simulink model "mdl_tubing_delays"  (R2020b)
settings: Solver=ode4  StartTime=0.0  StopTime=100  FixedStep=1e-3  RelTol=1e-3
undefined symbols (not defined in the file): m, n
libraries: simulink x2, sldelib x1, dspbuff3 x1
settings Model: EnablePacing=on  Creator=natha  LastModifiedBy=natha

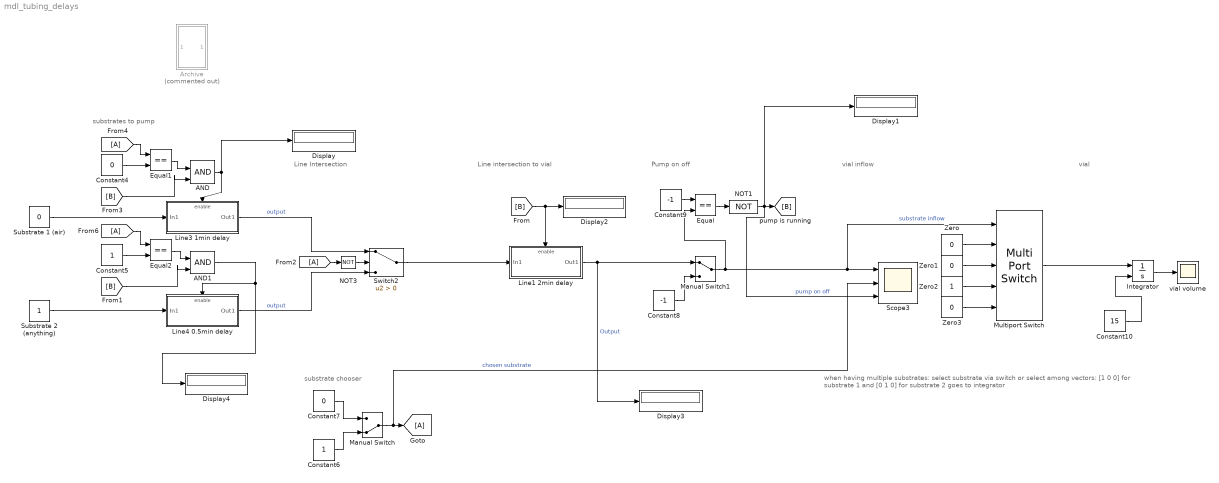
== system mdl_tubing_delays ==
  note: when having multiple substrates: select substrate via switch or select among vectors: [1 0 0] for substrate 1 and [0 1 0] for substrate 2 goes to integrator
  note: vial
  note: Line intersection to vial
  note: Pump on off
  note: substrate chooser
  note: Line Intersection
  note: substrates to pump
  note: vial inflow
  AND : Logic  IconShape=distinctive  AllPortsSameDT=off  OutDataTypeStr=boolean
  AND1 : Logic  IconShape=distinctive  AllPortsSameDT=off  OutDataTypeStr=boolean
  Archive : Subsystem  Commented=on
  Constant10 : Constant  Value=15
  Constant4 : Constant  Value=0
  Constant5 : Constant
  Constant6 : Constant
  Constant7 : Constant  Value=0
  Constant8 : Constant  Value=-1
  Constant9 : Constant  Value=-1
  Display{,1..4} (5 alike) : Display
  Equal : RelationalOperator  Operator===  OutDataTypeStr=boolean  RndMeth=Simplest
  Equal1 : RelationalOperator  Operator===  OutDataTypeStr=boolean  RndMeth=Simplest
  Equal2 : RelationalOperator  Operator===  OutDataTypeStr=boolean  RndMeth=Simplest
  Integrator : Integrator  InitialConditionSource=external
  Line1 2min delay : Subsystem  TreatAsAtomicUnit=on
  Line3 1min delay : Subsystem  TreatAsAtomicUnit=on
  Line4 0.5min delay : Subsystem  TreatAsAtomicUnit=on
  Manual Switch : ManualSwitch  CurrentSetting=0
  Manual Switch1 : ManualSwitch
  Multiport Switch : MultiPortSwitch  DataPortOrder=Specify indices  DataPortIndices={-1,0,1}  DataPortForDefault=Additional data port
  NOT1 : Logic  Operator=NOT  IconShape=distinctive  AllPortsSameDT=off  OutDataTypeStr=boolean
  NOT3 : Logic  Operator=NOT  IconShape=distinctive  AllPortsSameDT=off  OutDataTypeStr=boolean
  Scope3 : Scope  NumInputPorts=3
  Substrate 1 (air) : Constant  Value=0
  Substrate 2 (anything) : Constant
  Switch2 : Switch  Criteria=u2 > Threshold
  Zero : Constant  Value=0  OutDataTypeStr=Inherit: Inherit via back propagation
  Zero1 : Constant  Value=0  OutDataTypeStr=Inherit: Inherit via back propagation
  Zero2 : Constant  OutDataTypeStr=Inherit: Inherit via back propagation
  Zero3 : Constant  Value=0  OutDataTypeStr=Inherit: Inherit via back propagation
  vial volume : Scope
  wires:
  Line3 1min delay/1(Out1) -> Switch2/1  "output"
  Line4 0.5min delay/1(Out1) -> Switch2/3  "output"
  Constant6/1 -> Manual Switch/2
  Constant7/1 -> Manual Switch/1
  Manual Switch/1 -> Scope3/2, [A]  "chosen substrate"
  [A] -> NOT3/1
  Constant8/1 -> Manual Switch1/2
  Manual Switch1/1 -> Equal/2, Multiport Switch/1, Scope3/1  "substrate inflow"
  Constant9/1 -> Equal/1
  Equal/1 -> NOT1/1
  NOT1/1 -> Scope3/3, [B], Display1/1  "pump on off"
  [B] -> AND/2
  [A] -> Equal1/1
  Substrate 1 (air)/1 -> Line3 1min delay/1(In1)
  [B] -> Display2/1, Line1 2min delay/Enable
  Substrate 2 (anything)/1 -> Line4 0.5min delay/1(In1)
  Switch2/1 -> Line1 2min delay/1(In1)
  Line1 2min delay/1(Out1) -> Manual Switch1/1, Display3/1  "Output"
  AND/1 -> Line3 1min delay/Enable, Display/1
  [B] -> AND1/2
  AND1/1 -> Display4/1, Line4 0.5min delay/Enable
  NOT3/1 -> Switch2/2
  Equal1/1 -> AND/1
  Constant4/1 -> Equal1/2
  Constant5/1 -> Equal2/2
  Equal2/1 -> AND1/1
  [A] -> Equal2/1
  Zero/1 -> Multiport Switch/2
  Zero1/1 -> Multiport Switch/3
  Zero2/1 -> Multiport Switch/4
  Zero3/1 -> Multiport Switch/5
  Multiport Switch/1 -> Integrator/1
  Constant10/1 -> Integrator/2
  Integrator/1 -> vial volume/1

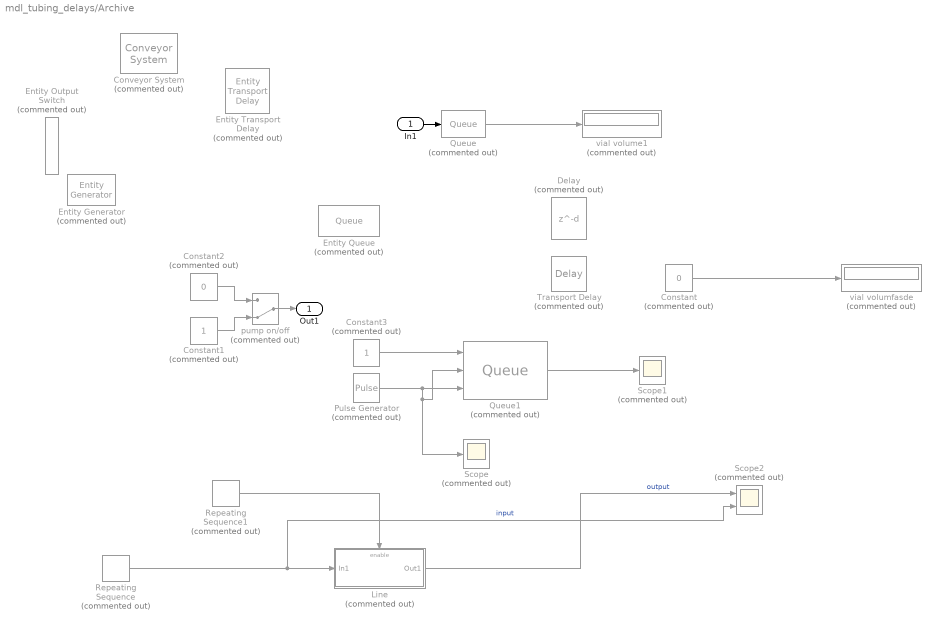
== system mdl_tubing_delays/Archive ==
  In1 : Inport
  Constant : Constant  Commented=on  Value=0
  Constant1 : Constant  Commented=on
  Constant2 : Constant  Commented=on  Value=0
  Constant3 : Constant  Commented=on
  Conveyor System : sldelib/Conveyor System  Commented=on  mConveyorLength=100  mConveyorSpeedSource=Dialog  mConveyorSpeed=1000  mInitialConveyorSpeed=1000  mMinDisBetEntity=0  mEntityLengthSource=Dialog  mEntityLength=1  mEntityLengthAttrName=Length  mOutputBlockedOpt=Accumulate  mErrorUponFullOpt=on  mNumEntitiesDepOpt=off  mNumEntitiesInBlockOpt=off  mEntityPendingOpt=off  mNumExtractedFromBlockOpt=off  mConveyorSpeedOpt=off
      settings: SourceProductBaseCode=SE
  Delay : Delay  Commented=on  DelayLengthSource=Input port  DelayLengthUpperLimit=1000000
      settings: InputPortMap=u0,p1
  Entity Output Switch : EntityOutputSwitch  Commented=on  InputPortMessageModes=m  OutputPortMessageModes=m,m  SwitchAttributeName=Attribute1
  Entity Transport Delay : EntityTransportDelay  Commented=on  InputPortMessageModes=m,n  OutputPortMessageModes=m
  Entity Generator : EntityGenerator  Commented=on  OutputPortMessageModes=m  EntityType=Structured  EntityTypeName=Entity
  Entity Queue : Queue  Commented=on  InputPortMessageModes=m  OutputPortMessageModes=m
  Line : Subsystem  Commented=on  TreatAsAtomicUnit=on
  Pulse Generator : DiscretePulseGenerator  Commented=on  PulseType=Time based  Period=10e-3  PulseWidth=10
  Queue : Queue  Commented=on  InputPortMessageModes=m  OutputPortMessageModes=m  OverwriteOldest=on  Capacity=16
  Queue1 : dspbuff3/Queue  Commented=on  depth=20  trigger=Rising edge  overflow=Dynamic reallocation  pes=Ignore  eso=off  fso=off  nso=off  clr=off  clrOutport=off  adf=on
      settings: SourceProductBaseCode=DS
  Repeating Sequence : simulink/Sources/Repeating Sequence  Commented=on  rep_seq_t=[0 2 2.001 4 4.001 6 6.001 7 7.001 10 10.001 100]  rep_seq_y=[-1 -1 2 2 0 0 3 3 1 1 -1 -1]
  Repeating Sequence1 : simulink/Sources/Repeating Sequence  Commented=on  rep_seq_t=[0 2]  rep_seq_y=[1 1]
  Scope : Scope  Commented=on
  Scope1 : Scope  Commented=on
  Scope2 : Scope  Commented=on  NumInputPorts=2
  Transport Delay : TransportDelay  Commented=on
  pump on/off : ManualSwitch  Commented=on  CurrentSetting=0
  vial volume1 : Display  Commented=on
  vial volumfasde : Display  Commented=on
  Out1 : Outport
  wires:
  Queue1/1 -> Scope1/1
  Constant/1 -> vial volumfasde/1
  Repeating Sequence/1 -> Scope2/2, Line/1(In1)  "input"
  In1/1 -> Queue/1
  Repeating Sequence1/1 -> Line/Enable
  Constant2/1 -> pump on/off/1
  Pulse Generator/1 -> Queue1/2, Queue1/3, Scope/1
  Constant1/1 -> pump on/off/2
  Queue/1 -> vial volume1/1
  Line/1(Out1) -> Scope2/1  "output"
  Constant3/1 -> Queue1/1
  pump on/off/1 -> Out1/1

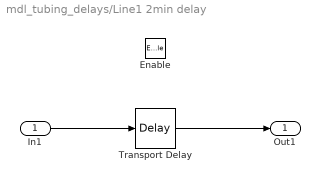
== system mdl_tubing_delays/Line1 2min delay ==
  In1 : Inport
  Enable : EnablePort
  Transport Delay : TransportDelay  DelayTime=2
  Out1 : Outport
  wires:
  Transport Delay/1 -> Out1/1
  In1/1 -> Transport Delay/1

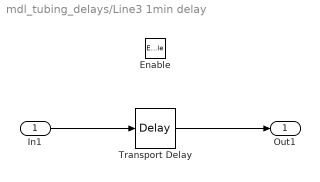
== system mdl_tubing_delays/Line3 1min delay ==
  In1 : Inport
  Enable : EnablePort
  Transport Delay : TransportDelay
  Out1 : Outport
  wires:
  In1/1 -> Transport Delay/1
  Transport Delay/1 -> Out1/1

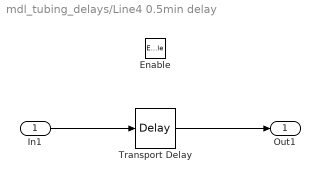
== system mdl_tubing_delays/Line4 0.5min delay ==
  In1 : Inport
  Enable : EnablePort
  Transport Delay : TransportDelay  DelayTime=0.5
  Out1 : Outport
  wires:
  Transport Delay/1 -> Out1/1
  In1/1 -> Transport Delay/1

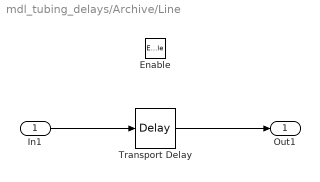
== system mdl_tubing_delays/Archive/Line ==
  In1 : Inport
  Enable : EnablePort
  Transport Delay : TransportDelay  DelayTime=0.5  InitialOutput=-1
  Out1 : Outport
  wires:
  In1/1 -> Transport Delay/1
  Transport Delay/1 -> Out1/1
